simulink model "w22_3"  (R2025b)
settings: Solver=ode4  StartTime=0.0  StopTime=30  FixedStep=1e-6  RelTol=1e-3
libraries: simulink_extras x5
settings Model: Creator=mmoha  LastModifiedBy=mmoha

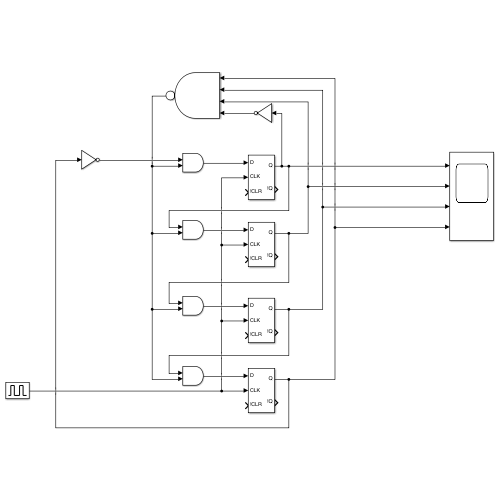
[thumbnail: Simulink's stored preview of the top-level diagram]
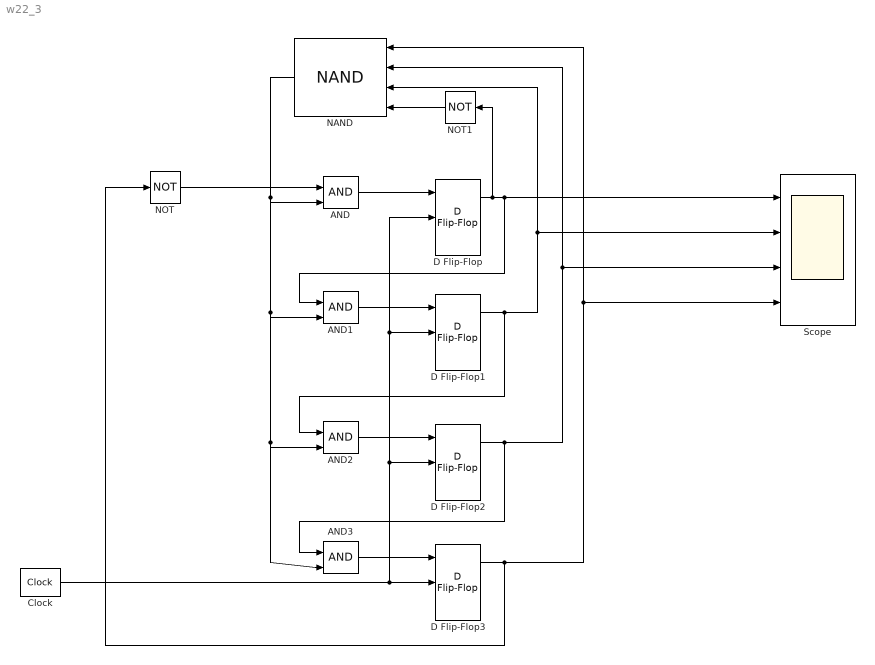
== system w22_3 ==
  AND{,1..3} (4 alike) : Logic  IconShape=distinctive  AllPortsSameDT=off  OutDataTypeStr=boolean
  Clock : simulink_extras/Flip Flops/Clock  period=2
  D Flip-Flop{,1..3} (4 alike) : simulink_extras/Flip Flops/D Flip-Flop
  NAND : Logic  Operator=NAND  Inputs=4  IconShape=distinctive  AllPortsSameDT=off  OutDataTypeStr=boolean
  NOT : Logic  Operator=NOT  IconShape=distinctive  AllPortsSameDT=off  OutDataTypeStr=boolean
  NOT1 : Logic  Operator=NOT  IconShape=distinctive  AllPortsSameDT=off  OutDataTypeStr=boolean
  Scope : Scope  NumInputPorts=4
      settings: ActiveDisplayYMinimum=-1  ActiveDisplayYMaximum=1
  wires:
  AND/1 -> D Flip-Flop/1
  AND1/1 -> D Flip-Flop1/1
  AND2/1 -> D Flip-Flop2/1
  AND3/1 -> D Flip-Flop3/1
  NOT/1 -> AND/1
  D Flip-Flop3/1 -> NOT/1, NAND/1, Scope/4
  D Flip-Flop/1 -> AND1/1, Scope/1, NOT1/1
  D Flip-Flop1/1 -> NAND/3, Scope/2, AND2/1
  D Flip-Flop2/1 -> AND3/1, NAND/2, Scope/3
  NOT1/1 -> NAND/4
  NAND/1 -> AND3/2, AND2/2, AND1/2, AND/2
  Clock/1 -> D Flip-Flop2/2, D Flip-Flop/2, D Flip-Flop1/2, D Flip-Flop3/2
